simulink model "justfuzzy"  (R2023a)
settings: Solver=VariableStepAuto  StartTime=0.0  StopTime=2  RelTol=1e-3
libraries: fuzblock x1
settings Model: Creator=mlean  LastModifiedBy=mlean

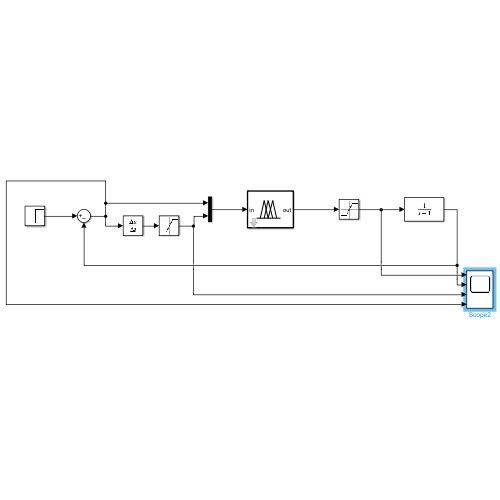
[thumbnail: Simulink's stored preview of the top-level diagram]
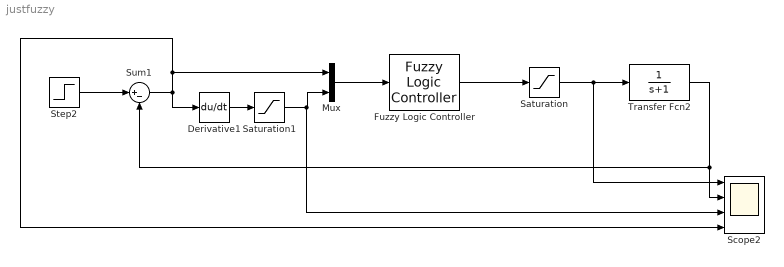
== system justfuzzy ==
  Derivative1 : Derivative  CoefficientInTFapproximation=0
  Fuzzy Logic Controller : fuzblock/Fuzzy Logic  Controller  FIS='man8.fis'  OutputSampleNumber=101  DataType=double  FuzzifiedInputs=off  RuleFiringStrengths=off  RuleOutputs=off  AggregatedOutputs=off  SimulateUsing=Interpreted execution  OutOfRangeInputValueMessage=warning  NoRuleFiredMessage=warning  EmptyOutputFuzzySetMessage=warning
  Mux : Mux  Inputs=2
  Saturation : Saturate  UpperLimit=10  LowerLimit=-10
  Saturation1 : Saturate  UpperLimit=10  LowerLimit=-10
  Scope2 : Scope  NumInputPorts=4
  Step2 : Step  Time=0  SampleTime=0
  Sum1 : Sum  Inputs=|+-
  Transfer Fcn2 : TransferFcn  Denominator=[1 1]
  wires:
  Sum1/1 -> Scope2/4, Mux/1, Derivative1/1
  Mux/1 -> Fuzzy Logic Controller/1
  Derivative1/1 -> Saturation1/1
  Fuzzy Logic Controller/1 -> Saturation/1
  Saturation1/1 -> Scope2/3, Mux/2
  Transfer Fcn2/1 -> Scope2/2, Sum1/2
  Saturation/1 -> Scope2/1, Transfer Fcn2/1
  Step2/1 -> Sum1/1
